simulink model "exe_1_1_a_sim"  (R2022b)
settings: Solver=VariableStepAuto  StartTime=0.0  StopTime=sim_T  RelTol=1e-3
values from neighbouring files (symbols this model uses):
  C = 1e-3    (= 0.001)    [exe_1_1.m]    (also in exe_1_3.m = [0 R])
  Ii = 10e-3    (= 0.01)    [exe_1_1.m]
  R = 1e-3    (= 0.001)    [exe_1_1.m]    (also in exe_1_3.m = 250)
settings Model: Creator=nicol  LastModifiedBy=nicol

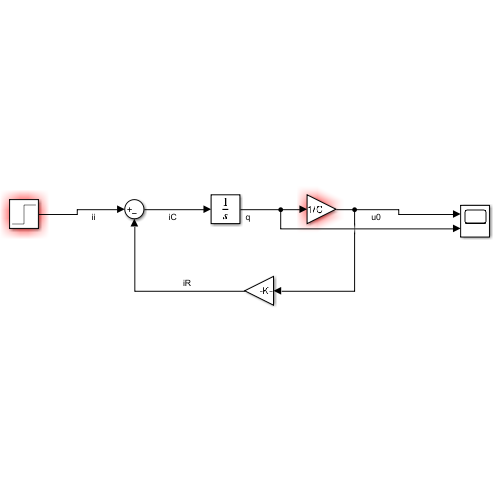
[thumbnail: Simulink's stored preview of the top-level diagram]
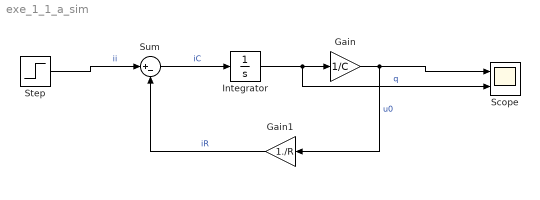
== system exe_1_1_a_sim ==
  Gain : Gain  Gain=1/C
  Gain1 : Gain  Gain=1./R
  Integrator : Integrator
  Scope : Scope  NumInputPorts=2
  Step : Step  Time=0  After=Ii  SampleTime=0
  Sum : Sum  Inputs=|+-
  wires:
  Integrator/1 -> Scope/2, Gain/1  "q"
  Gain/1 -> Gain1/1, Scope/1  "u0"
  Sum/1 -> Integrator/1  "iC"
  Gain1/1 -> Sum/2  "iR"
  Step/1 -> Sum/1  "ii"
